simulink model "lqr_2"  (R2020a)
settings: Solver=VariableStepAuto  StartTime=0.0  StopTime=inf  RelTol=1e-3
undefined symbols (not defined in the file): Angular, Linear, path
libraries: robotlib x4, simulink x1
settings Model: Creator=auvsl  LastModifiedBy=auvsl

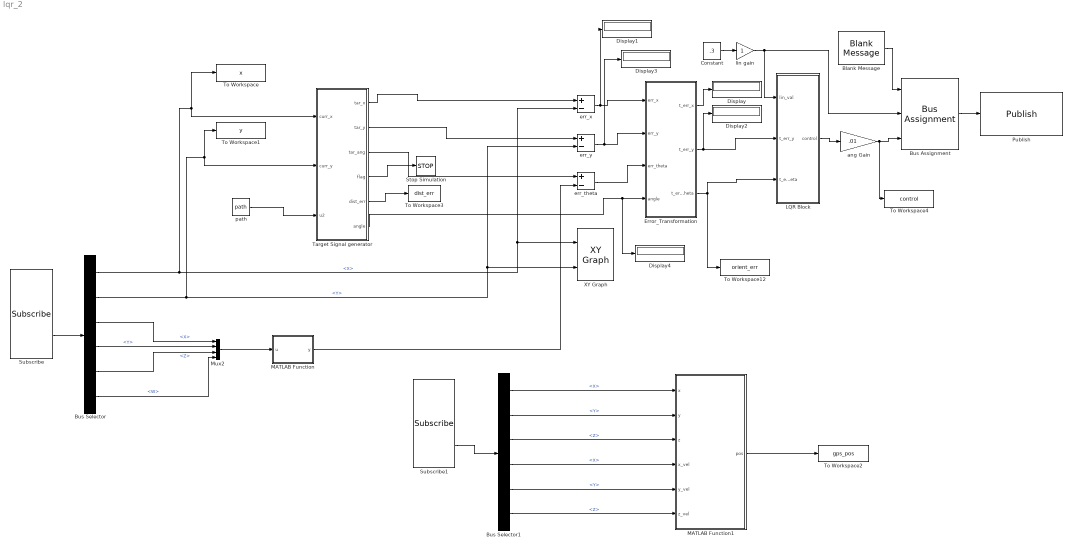
== system lqr_2 ==
  Blank Message : robotlib/Blank Message  messageClass=Message  entityType=geometry_msgs/Twist  messageType=geometry_msgs/Twist  SampleTime=inf
  Bus Assignment : BusAssignment  AssignedSignals=Linear.X,Angular.Z
  Bus Selector : BusSelector  OutputSignals=Pose.Pose.Position.X,Pose.Pose.Position.Y,Pose.Pose.Orientation.X,Pose.Pose.Orientation.Y,Pose.Pose.Orientation.Z,Pose.Pose.Orientation.W
  Bus Selector1 : BusSelector  OutputSignals=Pose.Pose.Position.X,Pose.Pose.Position.Y,Pose.Pose.Position.Z,Twist.Twist.Linear.X,Twist.Twist.Linear.Y,Twist.Twist.Linear.Z
  Constant : Constant  Value=.3
  Display{,1..4} (5 alike) : Display
  Error_Transformation : MATLAB Function  TreatAsAtomicUnit=on
  LQR Block : MATLAB Function  TreatAsAtomicUnit=on
  MATLAB Function : MATLAB Function  TreatAsAtomicUnit=on
  MATLAB Function1 : MATLAB Function  TreatAsAtomicUnit=on
  Mux2 : Mux
  Publish : robotlib/Publish  topicSource=Specify your own  topic=/rexrov/cmd_vel  messageType=geometry_msgs/Twist  messageQueueLength=1
  Stop Simulation : Stop
  Subscribe : robotlib/Subscribe  topicSource=Specify your own  topic=/rexrov/pose_gt  messageType=nav_msgs/Odometry  sampleTime=-1  messageQueueLength=1
  Subscribe1 : robotlib/Subscribe  topicSource=Specify your own  topic=/rexrov/pose_gt  messageType=nav_msgs/Odometry  sampleTime=-1  messageQueueLength=1
  Target Signal generator : MATLAB Function  TreatAsAtomicUnit=on
  To Workspace : ToWorkspace  VariableName=x  SampleTime=-1
  To Workspace1 : ToWorkspace  VariableName=y  SampleTime=-1
  To Workspace12 : ToWorkspace  VariableName=orient_err  SampleTime=-1
  To Workspace2 : ToWorkspace  VariableName=gps_pos  SampleTime=-1
  To Workspace3 : ToWorkspace  VariableName=dist_err  SampleTime=-1
  To Workspace4 : ToWorkspace  VariableName=control  SampleTime=-1
  XY Graph : simulink/Sinks/XY Graph  xmin=-25  xmax=25  ymin=-25  ymax=25  st=-1
  ang Gain : Gain  Gain=.01
  err_theta : Sum  Inputs=+-
  err_x : Sum  Inputs=+-
  err_y : Sum  Inputs=+-
  lin gain : Gain
  path : Constant  Value=path
  wires:
  Bus Selector/4 -> Mux2/2  "<Y>"
  Bus Selector/3 -> Mux2/1  "<X>"
  Subscribe/2 -> Bus Selector/1
  Bus Selector/5 -> Mux2/3  "<Z>"
  Bus Selector/6 -> Mux2/4  "<W>"
  Mux2/1 -> MATLAB Function/1(u)
  Bus Selector/1 -> XY Graph/1, err_x/2, To Workspace/1, Target Signal generator/1(curr_x)  "<X>"
  Bus Selector/2 -> XY Graph/2, err_y/2, To Workspace1/1, Target Signal generator/2(curr_y)  "<Y>"
  MATLAB Function/1(y) -> err_theta/2
  Bus Assignment/1 -> Publish/1
  Blank Message/1 -> Bus Assignment/1
  ang Gain/1 -> To Workspace4/1, Bus Assignment/3
  LQR Block/1(control) -> ang Gain/1
  lin gain/1 -> Bus Assignment/2, LQR Block/1(lin_val)
  Constant/1 -> lin gain/1
  err_y/1 -> Display3/1, Error_Transformation/2(err_y)
  Error_Transformation/2(t_err_y) -> Display2/1, LQR Block/2(t_err_y)
  Error_Transformation/3(t_err_theta) -> To Workspace12/1, LQR Block/3(t_err_theta)
  err_x/1 -> Display1/1, Error_Transformation/1(err_x)
  Target Signal generator/1(tar_x) -> err_x/1
  Target Signal generator/2(tar_y) -> err_y/1
  Target Signal generator/3(tar_ang) -> err_theta/1
  Target Signal generator/4(flag) -> Stop Simulation/1
  path/1 -> Target Signal generator/3(u2)
  err_theta/1 -> Error_Transformation/3(err_theta)
  Subscribe1/2 -> Bus Selector1/1
  Bus Selector1/1 -> MATLAB Function1/1(x)  "<X>"
  Bus Selector1/2 -> MATLAB Function1/2(y)  "<Y>"
  Bus Selector1/3 -> MATLAB Function1/3(z)  "<Z>"
  Bus Selector1/4 -> MATLAB Function1/4(x_vel)  "<X>"
  Bus Selector1/5 -> MATLAB Function1/5(y_vel)  "<Y>"
  Bus Selector1/6 -> MATLAB Function1/6(z_vel)  "<Z>"
  MATLAB Function1/1(pos) -> To Workspace2/1
  Target Signal generator/5(dist_err) -> To Workspace3/1
  Target Signal generator/6(angle) -> Display4/1, Error_Transformation/4(angle)
  Error_Transformation/1(t_err_x) -> Display/1

== matlab function lqr_2/LQR Block ==
  data: lin_val input; t_err_y input; control output; t_err_theta input
function control = fcn(lin_val,t_err_y,t_err_theta)

l=1.3; %length of vehicle
v=lin_val;
disp(v);

A=[0 -v;0 0];
B=[0 v/l]';


Q=[1100 0;0 1000];
R=[.001];

%k=lqr(A,B,Q,R);
k=[-1095.4 1001.1];

u=k*[t_err_y t_err_theta]';

control = u;

== matlab function lqr_2/Error_Transformation ==
  data: err_x input; t_err_x output; err_y input; err_theta input; t_err_y output; t_err_theta output; angle input
function [t_err_x,t_err_y,t_err_theta] = fcn(err_x,err_y,err_theta,angle)

% disp("ERROR IN X");
% disp(err_x);
% disp("ERROR IN Y");
% disp(err_y);
 disp("ERROR IN Theta");
 disp(err_theta);

if err_theta > 3.14
    err_theta=err_theta-2*3.14;
elseif err_theta<-3.14
    err_theta=err_theta+2*3.14;
end     

%theta_r=atan2(err_y,err_x);
theta_r=angle;
% disp("theta_r is");
% disp(theta_r);
mat=[-cos(theta_r) -sin(theta_r) 0;sin(theta_r) -cos(theta_r) 0;0 0 1];
% disp("transformation matrix is");
% disp(mat);
err_transformed=mat*[err_x err_y err_theta]' ;%transposed matrix

t_err_x=err_transformed(1);
t_err_y=err_transformed(2);
t_err_theta=err_transformed(3);


disp("Transformed ERROR IN X");
disp(t_err_x);
disp("Transformed ERROR IN Y");
disp(t_err_y);
disp("Transformed ERROR IN Theta");
disp(t_err_theta);

== matlab function lqr_2/Target Signal generator ==
  settings: updateMethod=DISCRETE
  data: curr_x input; curr_y input; tar_x output; u2 input; tar_y output; tar_ang output; flag output; dist_err output; angle output
function [tar_x,tar_y,tar_ang,flag,dist_err,angle] = fcn(curr_x,curr_y,u2)

persistent pathcount;
persistent pathlength;
persistent path;
persistent pathPre;


if isempty(pathcount)
   pathcount=1;
   pathPre=u2;
   [pathlength,~]=size(pathPre);  
   path=[pathPre; pathPre(pathlength,1)+100 pathPre(pathlength,2)+100]; %sim takes multiple iterations to stop after reaching final point, so this prevents it from breaking
end

pos=[curr_x curr_y]; % [x,y] 
target=path(pathcount+1,:);
past=path(pathcount,:);



tar_x = target(1);
tar_y = target(2);

past_x=past(1);
past_y=past(2);

angle = atan2(tar_y-past_y,tar_x-past_x);

tar_ang=atan2(tar_y-past_y,tar_x-past_x);


%Distance Error calculation

a1=curr_x*(past_y-tar_y);
a2=curr_y*(tar_x-past_x);
a3=tar_y*past_x-tar_x*past_y;
a=-(a1+a2+a3);

b=norm([(past_y-tar_y) (past_x-tar_x)]);
dist_err=a/b;

%err=
if ((power(power(tar_x-curr_x,2)+power(tar_y-curr_y,2),.5) <=.2)) %this is the line that must have an additional thetaFinal condition added
    pathcount=pathcount+1;
end

flag=0;
if (pathcount==pathlength)
    flag=1;
end

a=mod(pathcount,2)+1;

== matlab function lqr_2/MATLAB Function1 ==
  data: x input; pos output; y input; z input; x_vel input; y_vel input; z_vel input
function pos = fcn(x,y,z,x_vel,y_vel,z_vel)

% fs = 1;
% duration = 1000;
% numSamples = duration*fs;
%numSamples = 2;

%refLoc = [42.2825 -71.343 53.0352];
% refLoc = [1 1 20]; %replace this with current location

refLoc = [0 0 20];

% truePosition = zeros(numSamples,3); %replace this with current position
% trueVelocity = zeros(numSamples,3); %replace this with current velocity

%gps = gpsSensor('SampleRate',fs,'ReferenceLocation',refLoc);
gps = gpsSensor('ReferenceLocation',refLoc);

truePosition = [x,y,z];
trueVelocity = [x_vel,y_vel,z_vel];

position = gps(truePosition,trueVelocity);

% 
% t = (0:(numSamples-1))/fs;
% 
% subplot(3, 1, 1)
% plot(t, position(:,1), ...
%      t, ones(numSamples)*refLoc(1))
% title('GPS Sensor Readings')
% ylabel('Latitude (degrees)')
% 
% subplot(3, 1, 2)
% plot(t, position(:,2), ...
%      t, ones(numSamples)*refLoc(2))
% ylabel('Longitude (degrees)')
% 
% subplot(3, 1, 3)
% plot(t, position(:,3), ...
%      t, ones(numSamples)*refLoc(3))
% ylabel('Altitude (m)')
% xlabel('Time (s)')
% 



pos = position;

== matlab function lqr_2/MATLAB Function ==
  data: u input; y output
function y = fcn(u)
quat = [u(1) u(2) u(3) u(4)];
euler = quat2eul(quat);
yaw = euler(3);
y = yaw;
